simulink model "gm_sampleModel1933_1_sub"  (R2023a)
settings: Solver=VariableStepAuto  StartTime=0.0  StopTime=10.0  RelTol=1e-3
libraries: simulink x2
settings Model: Creator=user1  LastModifiedBy=user1
settings OptimizationCC: BlockReduction=off  ConditionallyExecuteInputs=off
settings DebuggingCC: InheritedTsInSrcMsg=none

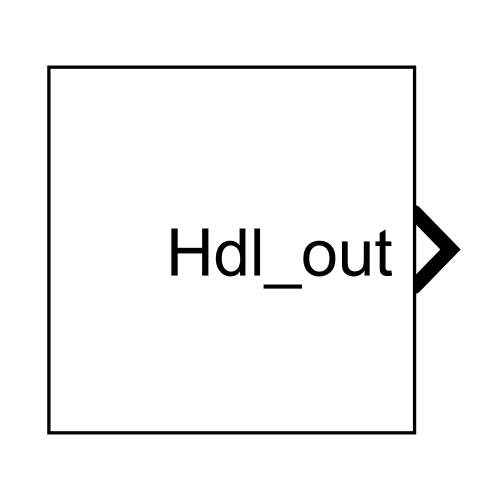
[thumbnail: Simulink's stored preview of the top-level diagram]
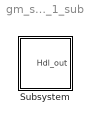
== system gm_sampleModel1933_1_sub ==
  Subsystem : Subsystem

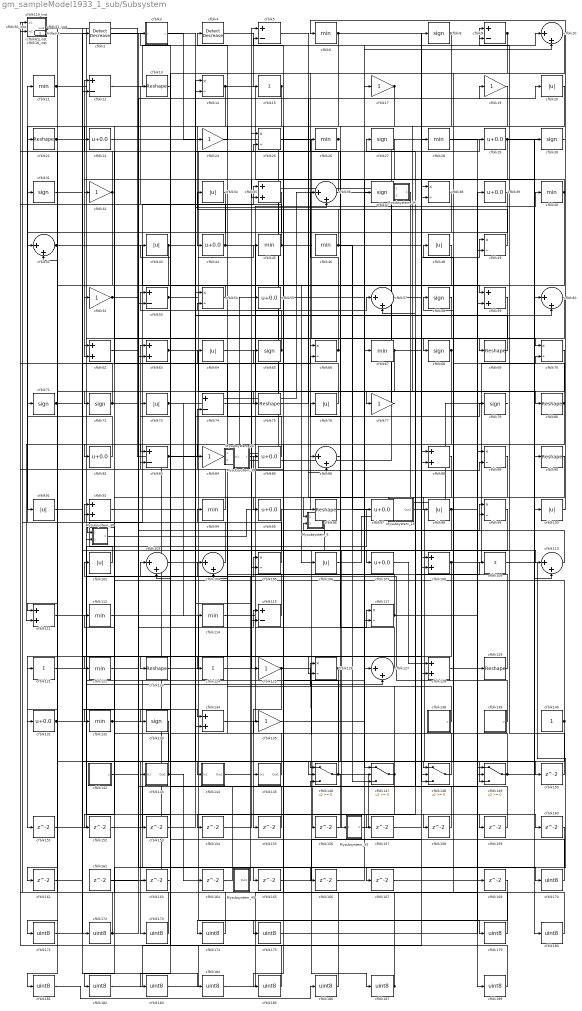
== system gm_sampleModel1933_1_sub/Subsystem ==
  Mysubsystem_13 : Subsystem
  Mysubsystem_24 : Subsystem
  Mysubsystem_30 : Subsystem
  Mysubsystem_33 : Subsystem
  Mysubsystem_34 : Subsystem
  Mysubsystem_39 : Subsystem
  Mysubsystem_45 : Subsystem
  Mysubsystem_9 : Subsystem
  cfblk{10,36,41,57,60,86,103..104,110,127} (10 alike) : Sum  Inputs=|++  OutDataTypeStr=uint8
  cfblk{20,34,43,48,64,73,76,91,98,100,102,106} (12 alike) : Abs  OutDataTypeStr=uint8  SaturateOnIntegerOverflow=off
  cfblk{14,25,38,49,54,66,70,89,99,105,117,126} (12 alike) : Product  Inputs=*/  OutDataTypeStr=uint8  RndMeth=Zero  SaturateOnIntegerOverflow=on
  cfblk{22,29,39,44,55,82,85,95,97,107,131} (11 alike) : Bias  Bias=0.0  SaturateOnIntegerOverflow=off
  cfblk{35,59,62..63,88,92,108,111,128,134} (10 alike) : Sum  OutDataTypeStr=uint8
  cfblk{15,109,121,124} (4 alike) : Sum  Inputs=+  OutDataTypeStr=uint8
  cfblk{6,11,26,28,40,45..46,67,94,112,114,122,132} (13 alike) : MinMax  OutDataTypeStr=uint8
  cfblk113_inst : Subsystem
  cfblk{5,9,12,53,74,83,115} (7 alike) : Sum  Inputs=+-  OutDataTypeStr=uint8
  cfblk119_inst : Subsystem
  cfblk{13,21,69,75,80,90,96,123,129} (9 alike) : Reshape
  cfblk{17,19,24,32,52,77,84,125,135} (9 alike) : Gain  OutDataTypeStr=uint8
  cfblk{8,27,30..31,37,58,65,68,71..72,79,133} (12 alike) : Signum
  cfblk138 : Subsystem  mask(Counter Free-Running){NumBits=double(16), tsamp=double(-1)}
      mask prompts: NumBits "Simulink:masks:NumberOfBits_MP"; tsamp "Simulink:masks:SampleTime_MP"
      mask help: Simulink:masks:CounterFreeRunning_MD
  cfblk139 : Subsystem  mask(Counter Limited){uplimit=double(7), tsamp=double(-1)}
      mask prompts: uplimit "Simulink:masks:UpperLimit_MP"; tsamp "Simulink:masks:SampleTime_MP"
      mask help: Simulink:masks:CounterLimited_MD
      mask init:
      | nbits = double(8);
      | tsamp = double(-1);
      | uplimit = double(7);
  cfblk140 : Constant  OutDataTypeStr=uint8  SampleTime=-1
  cfblk142 : Subsystem  mask(Counter Limited){uplimit=double(7), tsamp=double(-1)}
      mask prompts: uplimit "Simulink:masks:UpperLimit_MP"; tsamp "Simulink:masks:SampleTime_MP"
      mask help: Simulink:masks:CounterLimited_MD
      mask init:
      | nbits = double(8);
      | tsamp = double(-1);
      | uplimit = double(7);
  cfblk143 : Subsystem
  cfblk144 : Subsystem
  cfblk145 : Subsystem
  cfblk{146..149} (4 alike) : Switch  OutDataTypeStr=uint8  SaturateOnIntegerOverflow=off  InputSameDT=off
  cfblk{150..167,169} (19 alike) : Delay  SampleTime=1
  cfblk16_inst : Subsystem
  cfblk{170..175,179..187,189} (16 alike) : DataTypeConversion  OutDataTypeStr=uint8  SaturateOnIntegerOverflow=off  RndMeth=Floor
  cfblk2 : simulink/Logic and Bit Operations/Detect Decrease  vinit=0.0  OutDataTypeStr=uint8
      settings: LibrarySourceBlock=|
      | hdlsllib/Logic and Bit
      | Operations/Detect
      | Decrease
  cfblk3 : Subsystem  mask(Compare To Constant){relop=<=, const=double(3), OutDataTypeStr=uint8, ZeroCross=on}
      mask prompts: relop "Simulink:masks:Operator_MP"; const "Simulink:masks:ConstantValue_MP"; OutDataTypeStr "Simulink:masks:OutputDataType_MP"; ZeroCross "Simulink:masks:EnableZerocrossingDetection_MP"
      mask help: Simulink:masks:CompareToConstant_MD
      mask init:
      | OutDataTypeStr = 'uint8';
      | ZeroCross = 'on';
      | blkName = 'sampleModel1933_1_sub/Subsystem/cfblk3';
      | const = double(3);
      | const_str = '3.0';
      | const_val = double(3);
      | relop = '<=';
      | setValue = 'fixdt(0, 8)';
      | str = '<= 3';
      mask TypeOptions relop: == | ~= | < | <= | >= | >
      mask TypeOptions OutDataTypeStr: Simulink:masks:uint8 | Simulink:masks:boolean
      mask Callback ZeroCross: sl('zeroCrossEnable', gcbh);
      mask Display: disp(str)
  cfblk4 : simulink/Logic and Bit Operations/Detect Decrease  vinit=0.0  OutDataTypeStr=uint8
      settings: LibrarySourceBlock=|
      | hdlsllib/Logic and Bit
      | Operations/Detect
      | Decrease
  cfblk50_inst : Subsystem
  cfblk51_inst : Subsystem
  cfblk61_inst : Subsystem
  Hdl_out : Outport  OutDataTypeStr=uint8  SampleTime=1
  wires:
  Mysubsystem_13/1(Out1) -> cfblk150/1
  Mysubsystem_24/1(Out1) -> cfblk162/1
  Mysubsystem_30/1(Out1) -> Mysubsystem_13/2(In2)
  Mysubsystem_33/1(Out1) -> cfblk158/1
  Mysubsystem_34/1(Out1) -> Mysubsystem_9/1(In1)
  Mysubsystem_39/1(Y) -> cfblk57/1
  Mysubsystem_45/1(Out1) -> cfblk103/1
  Mysubsystem_9/1(Out1) -> Mysubsystem_33/1(In1)
  cfblk10/1 -> cfblk96/1
  cfblk100/1 -> cfblk6/1
  cfblk102/1 -> cfblk35/1
  cfblk103/1 -> cfblk187/1
  cfblk104/1 -> cfblk11/1
  cfblk105/1 -> cfblk16_inst/1(in1)
  cfblk106/1 -> Mysubsystem_13/3(In3)
  cfblk107/1 -> cfblk128/1
  cfblk108/1 -> cfblk70/2, cfblk151/1
  cfblk109/1 -> cfblk167/1
  cfblk11/1 -> cfblk128/2, cfblk127/2, cfblk159/1
  cfblk110/1 -> Mysubsystem_9/2(In2)
  cfblk111/1 -> cfblk123/1
  cfblk112/1 -> cfblk179/1
  cfblk113_inst/1(out1) -> cfblk68/1
  cfblk114/1 -> cfblk40/1
  cfblk115/1 -> cfblk51_inst/1(in1)
  cfblk117/1 -> cfblk63/1, cfblk189/1
  cfblk119_inst/1(out1) -> Mysubsystem_30/2(In2)
  cfblk12/1 -> cfblk10/1
  cfblk121/1 -> cfblk97/1
  cfblk122/1 -> cfblk99/1
  cfblk123/1 -> cfblk29/1
  cfblk124/1 -> cfblk117/1
  cfblk125/1 -> cfblk156/1, cfblk155/1
  cfblk126/1 -> cfblk173/1, cfblk161/1
  cfblk127/1 -> cfblk76/1
  cfblk128/1 -> cfblk59/2
  cfblk129/1 -> cfblk27/1
  cfblk13/1 -> cfblk163/1
  cfblk131/1 -> cfblk149/3, cfblk104/1, cfblk105/1
  cfblk132/1 -> cfblk37/1, cfblk165/1
  cfblk133/1 -> cfblk143/1(In1)
  cfblk134/1 -> cfblk109/1
  cfblk135/1 -> cfblk17/1
  cfblk138/1(y) -> cfblk126/1
  cfblk139/1(y) -> cfblk102/1
  cfblk14/1 -> cfblk127/1, cfblk110/2, cfblk122/1
  cfblk140/1 -> cfblk92/1, cfblk145/1(In1)
  cfblk142/1(y) -> cfblk115/1
  cfblk143/1(Out1) -> cfblk92/2, cfblk164/1
  cfblk144/1(Out1) -> cfblk89/2
  cfblk145/1(Out1) -> cfblk135/1
  cfblk146/1 -> cfblk25/2, cfblk160/1
  cfblk147/1 -> cfblk74/2, cfblk154/1
  cfblk148/1 -> cfblk94/1
  cfblk149/1 -> cfblk30/1, cfblk3/1(u)
  cfblk15/1 -> cfblk62/2, cfblk44/1, cfblk84/1
  cfblk150/1 -> cfblk9/1
  cfblk151/1 -> cfblk14/1
  cfblk152/1 -> cfblk108/1
  cfblk153/1 -> cfblk36/2
  cfblk154/1 -> cfblk99/2
  cfblk155/1 -> cfblk54/2
  cfblk156/1 -> cfblk147/2
  cfblk157/1 -> cfblk49/1
  cfblk158/1 -> cfblk83/2
  cfblk159/1 -> cfblk57/2
  cfblk16_inst/1(out1) -> cfblk108/2
  cfblk160/1 -> cfblk182/1
  cfblk161/1 -> cfblk66/2
  cfblk162/1 -> cfblk63/2
  cfblk163/1 -> cfblk53/1
  cfblk164/1 -> cfblk149/1
  cfblk165/1 -> cfblk88/2
  cfblk166/1 -> cfblk10/2
  cfblk167/1 -> cfblk89/1
  cfblk169/1 -> cfblk174/1
  cfblk17/1 -> cfblk91/1, cfblk86/1
  cfblk170/1 -> cfblk73/1
  cfblk171/1 -> cfblk2/1
  cfblk172/1 -> cfblk16_inst/2(in2), cfblk146/3, cfblk119_inst/2(in2)
  cfblk173/1 -> cfblk31/1
  cfblk174/1 -> cfblk113_inst/2(in2)
  cfblk175/1 -> cfblk169/1
  cfblk179/1 -> cfblk58/1
  cfblk180/1 -> cfblk112/1
  cfblk181/1 -> cfblk186/1
  cfblk182/1 -> cfblk38/1
  cfblk183/1 -> cfblk38/2
  cfblk184/1 -> cfblk49/2
  cfblk185/1 -> cfblk50_inst/1(in1)
  cfblk186/1 -> cfblk50_inst/2(in2)
  cfblk187/1 -> cfblk85/1, cfblk71/1, cfblk61_inst/1(in1)
  cfblk189/1 -> cfblk103/2
  cfblk19/1 -> cfblk75/1
  cfblk2/1 -> cfblk170/1
  cfblk20/1 -> cfblk24/1
  cfblk21/1 -> cfblk180/1, cfblk66/1
  cfblk22/1 -> cfblk110/1
  cfblk24/1 -> cfblk4/1
  cfblk25/1 -> cfblk59/1
  cfblk26/1 -> Hdl_out/1, Mysubsystem_24/1(In1)
  cfblk27/1 -> cfblk62/1
  cfblk28/1 -> cfblk80/1
  cfblk29/1 -> cfblk60/1, cfblk35/2
  cfblk3/1(y) -> cfblk115/2
  cfblk30/1 -> Mysubsystem_24/2(In2)
  cfblk31/1 -> cfblk172/1
  cfblk32/1 -> cfblk61_inst/2(in2), cfblk111/1
  cfblk34/1 -> cfblk131/1
  cfblk35/1 -> cfblk152/1
  cfblk36/1 -> cfblk12/1
  cfblk37/1 -> cfblk74/1
  cfblk38/1 -> cfblk181/1
  cfblk39/1 -> cfblk41/1
  cfblk4/1 -> cfblk15/1
  cfblk40/1 -> cfblk53/2, cfblk32/1
  cfblk41/1 -> cfblk148/3, cfblk106/1
  cfblk43/1 -> cfblk14/2, Mysubsystem_30/1(In1)
  cfblk44/1 -> cfblk113_inst/1(in1), cfblk117/2
  cfblk45/1 -> cfblk90/1, cfblk86/2, cfblk13/1
  cfblk46/1 -> cfblk5/2, cfblk147/3, cfblk28/1
  cfblk48/1 -> cfblk153/1
  cfblk49/1 -> cfblk34/1
  cfblk5/1 -> cfblk147/1
  cfblk50_inst/1(out1) -> cfblk184/1
  cfblk51_inst/1(out1) -> cfblk144/1(In1), Mysubsystem_39/1(In1)
  cfblk52/1 -> cfblk82/1, cfblk149/2
  cfblk53/1 -> cfblk146/1, cfblk45/1
  cfblk54/1 -> cfblk52/1
  cfblk55/1 -> cfblk67/1
  cfblk57/1 -> cfblk69/1
  cfblk58/1 -> cfblk72/1
  cfblk59/1 -> cfblk157/1
  cfblk6/1 -> cfblk88/1, cfblk171/1
  cfblk60/1 -> cfblk148/1
  cfblk61_inst/1(out1) -> cfblk41/2, cfblk126/2
  cfblk62/1 -> cfblk166/1
  cfblk63/1 -> cfblk100/1, cfblk70/1
  cfblk64/1 -> cfblk129/1
  cfblk65/1 -> cfblk5/1, cfblk43/1
  cfblk66/1 -> cfblk36/1, cfblk146/2
  cfblk67/1 -> cfblk8/1, cfblk105/2
  cfblk68/1 -> cfblk185/1, cfblk175/1
  cfblk69/1 -> cfblk54/1
  cfblk70/1 -> cfblk121/1
  cfblk71/1 -> cfblk134/1, cfblk107/1
  cfblk72/1 -> cfblk51_inst/2(in2), cfblk19/1
  cfblk73/1 -> Mysubsystem_34/1(In1), cfblk114/1
  cfblk74/1 -> cfblk125/1
  cfblk75/1 -> cfblk20/1
  cfblk76/1 -> cfblk22/1
  cfblk77/1 -> Mysubsystem_34/2(In2)
  cfblk79/1 -> Mysubsystem_13/1(In1)
  cfblk8/1 -> cfblk134/2, cfblk77/1
  cfblk80/1 -> cfblk48/1, cfblk111/2
  cfblk82/1 -> cfblk21/1
  cfblk83/1 -> cfblk65/1, cfblk60/2, cfblk25/1
  cfblk84/1 -> cfblk55/1
  cfblk85/1 -> cfblk64/1
  cfblk86/1 -> cfblk26/1
  cfblk88/1 -> cfblk132/1
  cfblk89/1 -> cfblk124/1
  cfblk9/1 -> cfblk98/1, cfblk83/1, cfblk148/2
  cfblk90/1 -> cfblk95/1
  cfblk91/1 -> cfblk12/2
  cfblk92/1 -> cfblk79/1
  cfblk94/1 -> cfblk119_inst/1(in1)
  cfblk95/1 -> cfblk133/1
  cfblk96/1 -> cfblk9/2
  cfblk97/1 -> cfblk46/1
  cfblk98/1 -> cfblk39/1, cfblk104/2
  cfblk99/1 -> cfblk183/1

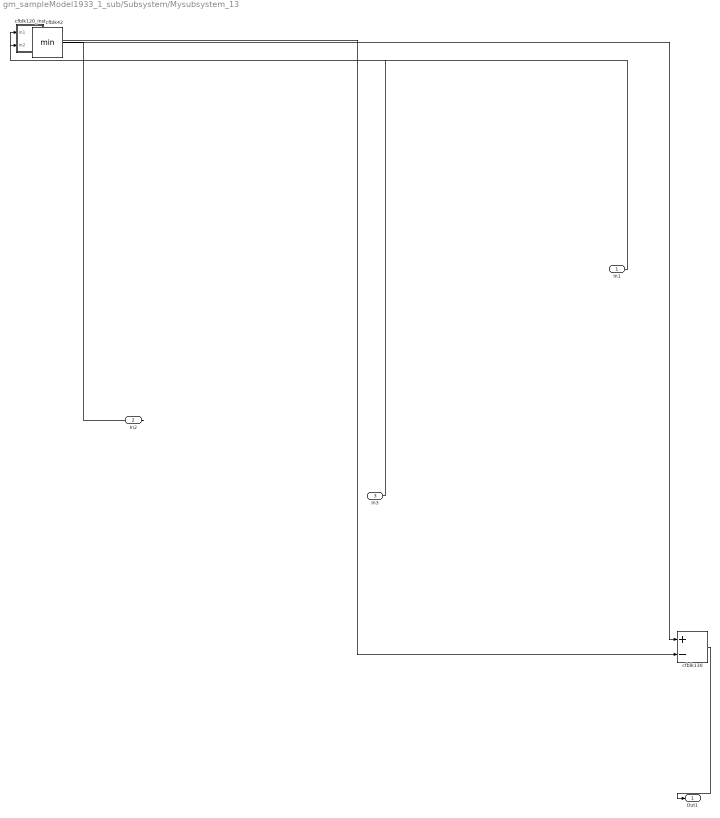
== system gm_sampleModel1933_1_sub/Subsystem/Mysubsystem_13 ==
  In1 : Inport  OutDataTypeStr=uint8  PortDimensions=1  SampleTime=1
  In2 : Inport  Port=2  OutDataTypeStr=uint8  PortDimensions=1  SampleTime=1
  In3 : Inport  Port=3  OutDataTypeStr=uint8  PortDimensions=1  SampleTime=1
  cfblk120_inst : Subsystem
  cfblk130 : Sum  Inputs=+-
  cfblk42 : MinMax
  Out1 : Outport  SampleTime=1
  wires:
  In1/1 -> cfblk120_inst/1(in1)
  In2/1 -> cfblk42/1
  In3/1 -> cfblk120_inst/2(in2)
  cfblk120_inst/1(out1) -> cfblk130/2
  cfblk130/1 -> Out1/1
  cfblk42/1 -> cfblk130/1

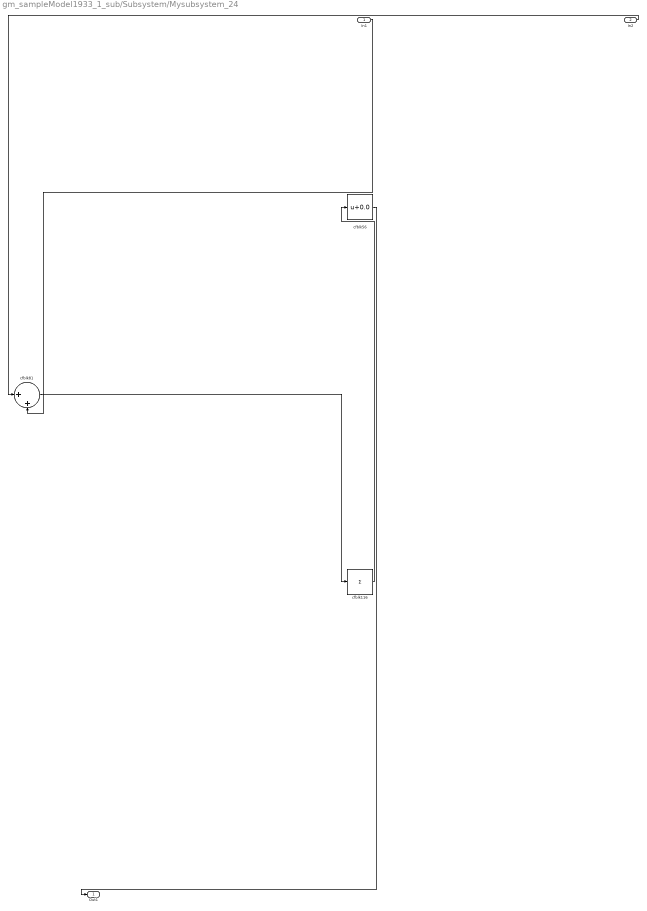
== system gm_sampleModel1933_1_sub/Subsystem/Mysubsystem_24 ==
  In1 : Inport  OutDataTypeStr=uint8  PortDimensions=1  SampleTime=1
  In2 : Inport  Port=2  OutDataTypeStr=uint8  PortDimensions=1  SampleTime=1
  cfblk116 : Sum  Inputs=+
  cfblk56 : Bias  Bias=0.0  SaturateOnIntegerOverflow=off
  cfblk81 : Sum  Inputs=|++
  Out1 : Outport  SampleTime=1
  wires:
  In1/1 -> cfblk81/2
  In2/1 -> cfblk81/1
  cfblk116/1 -> cfblk56/1
  cfblk56/1 -> Out1/1
  cfblk81/1 -> cfblk116/1

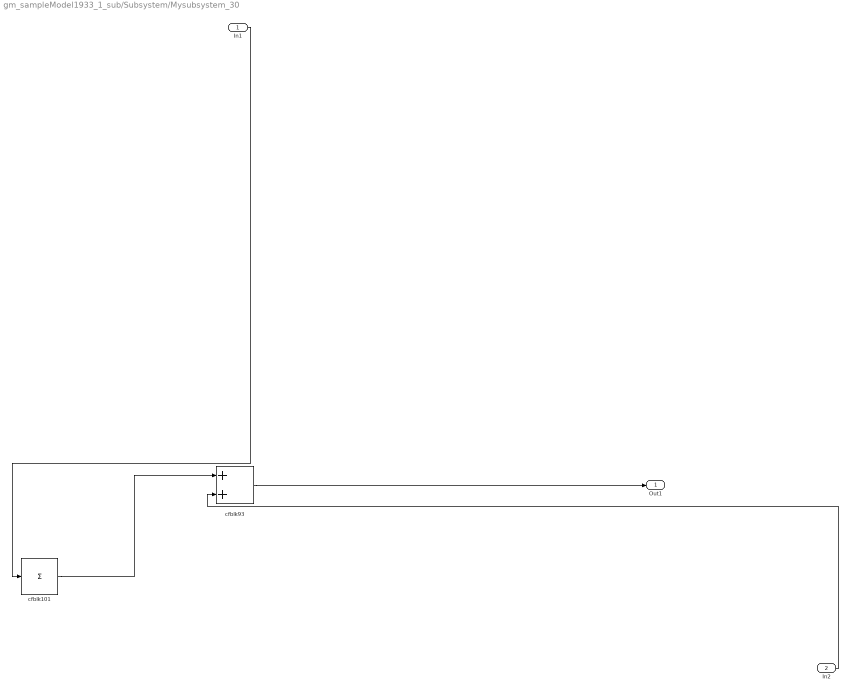
== system gm_sampleModel1933_1_sub/Subsystem/Mysubsystem_30 ==
  In1 : Inport  OutDataTypeStr=uint8  PortDimensions=1  SampleTime=1
  In2 : Inport  Port=2  OutDataTypeStr=uint8  PortDimensions=1  SampleTime=1
  cfblk101 : Sum  Inputs=+
  cfblk93 : Sum
  Out1 : Outport  SampleTime=1
  wires:
  In1/1 -> cfblk101/1
  In2/1 -> cfblk93/2
  cfblk101/1 -> cfblk93/1
  cfblk93/1 -> Out1/1

== system gm_sampleModel1933_1_sub/Subsystem/Mysubsystem_33 ==
  In1 : Inport  OutDataTypeStr=uint16  PortDimensions=1  SampleTime=1
  cfblk176 : DataTypeConversion  SaturateOnIntegerOverflow=off  RndMeth=Floor
  Out1 : Outport  SampleTime=1
  wires:
  In1/1 -> cfblk176/1
  cfblk176/1 -> Out1/1

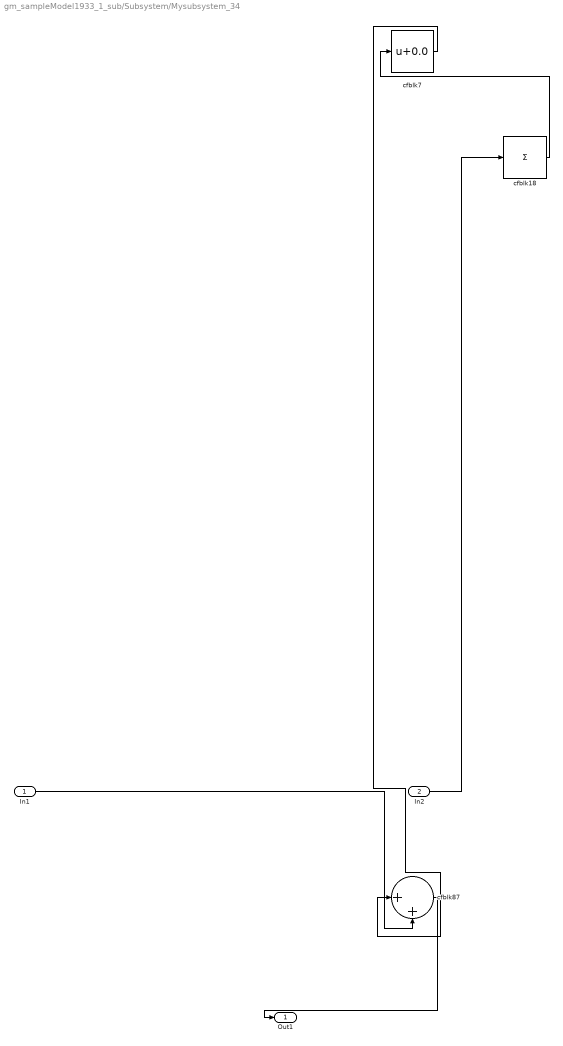
== system gm_sampleModel1933_1_sub/Subsystem/Mysubsystem_34 ==
  In1 : Inport  OutDataTypeStr=uint8  PortDimensions=1  SampleTime=1
  In2 : Inport  Port=2  OutDataTypeStr=uint8  PortDimensions=1  SampleTime=1
  cfblk18 : Sum  Inputs=+
  cfblk7 : Bias  Bias=0.0  SaturateOnIntegerOverflow=off
  cfblk87 : Sum  Inputs=|++
  Out1 : Outport  SampleTime=1
  wires:
  In1/1 -> cfblk87/2
  In2/1 -> cfblk18/1
  cfblk18/1 -> cfblk7/1
  cfblk7/1 -> cfblk87/1
  cfblk87/1 -> Out1/1

== system gm_sampleModel1933_1_sub/Subsystem/Mysubsystem_39 ==
  In1 : Inport  OutDataTypeStr=uint8  PortDimensions=1  SampleTime=1
  cfblk1 : Subsystem  mask(Detect Rise Positive){vinit=double(0), InputProcessing=Elements as channels (sample based), OutDataTypeStr=boolean}
      mask prompts: vinit "Simulink:masks:InitialCondition_MP"; InputProcessing "Simulink:masks:InputProcessing_MP"; OutDataTypeStr "Simulink:masks:OutputDataType_MP"
      mask help: Simulink:masks:DetectRisePositive_MD
      mask init:
      | InputProcessing = 'Elements as channels (sample based)';
      | OutDataTypeStr = 'boolean';
      | vinit = double(0);
      mask TypeOptions InputProcessing: Simulink:masks:ColumnsAsChannelsFrameBased | Simulink:masks:ElementsAsChannelsSampleBased
      mask TypeOptions OutDataTypeStr: Simulink:masks:uint8 | Simulink:masks:boolean
      mask Display: fprintf('U > 0\n&  NOT\nU/z > 0')
  cfblk168 : Delay  SampleTime=1
  Y : Outport  SampleTime=1
  wires:
  In1/1 -> cfblk168/1
  cfblk1/1(Y) -> Y/1
  cfblk168/1 -> cfblk1/1(U)

== system gm_sampleModel1933_1_sub/Subsystem/Mysubsystem_45 ==
  cfblk141 : Ground
  cfblk188 : DataTypeConversion  OutDataTypeStr=uint8  SaturateOnIntegerOverflow=off  RndMeth=Floor
  Out1 : Outport  SampleTime=1
  wires:
  cfblk141/1 -> cfblk188/1
  cfblk188/1 -> Out1/1

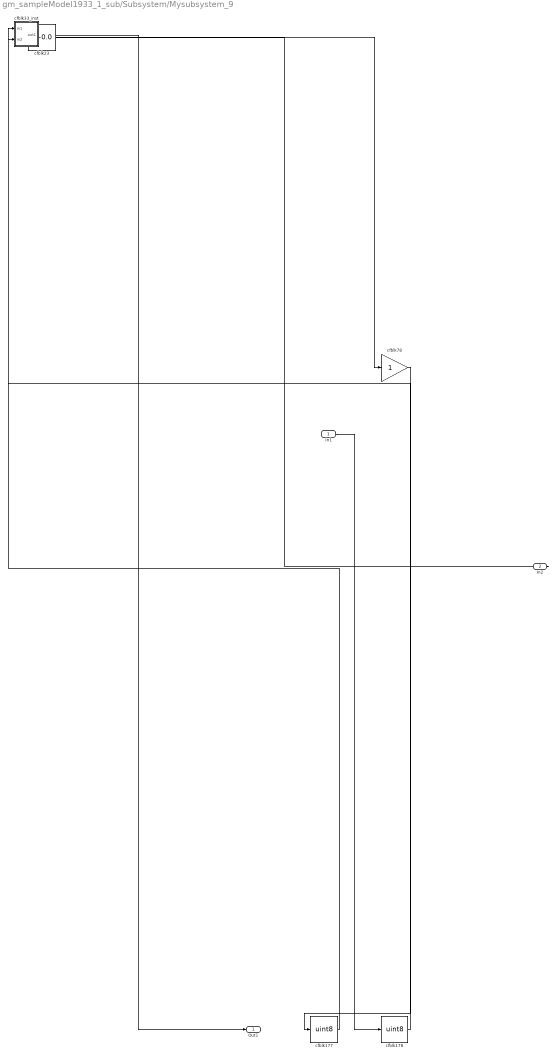
== system gm_sampleModel1933_1_sub/Subsystem/Mysubsystem_9 ==
  In1 : Inport  OutDataTypeStr=uint8  PortDimensions=1  SampleTime=1
  In2 : Inport  Port=2  OutDataTypeStr=uint8  PortDimensions=1  SampleTime=1
  cfblk177 : DataTypeConversion  OutDataTypeStr=uint8  SaturateOnIntegerOverflow=off  RndMeth=Floor
  cfblk178 : DataTypeConversion  OutDataTypeStr=uint8  SaturateOnIntegerOverflow=off  RndMeth=Floor
  cfblk23 : Bias  Bias=0.0  SaturateOnIntegerOverflow=off
  cfblk33_inst : Subsystem
  cfblk78 : Gain
  Out1 : Outport  SampleTime=1
  wires:
  In1/1 -> cfblk178/1
  In2/1 -> cfblk23/1
  cfblk177/1 -> cfblk33_inst/1(in1)
  cfblk178/1 -> cfblk33_inst/2(in2)
  cfblk23/1 -> cfblk78/1
  cfblk33_inst/1(out1) -> Out1/1
  cfblk78/1 -> cfblk177/1

== system gm_sampleModel1933_1_sub/Subsystem/cfblk113_inst ==
  in1 : Inport  OutDataTypeStr=uint8  SampleTime=1
  in2 : Inport  Port=2  OutDataTypeStr=uint8  SampleTime=1
  mul_cfblk113_dotp_mulcomp : Product  Inputs=**  OutDataTypeStr=uint8  SampleTime=1
  out1 : Outport  OutDataTypeStr=uint8  SampleTime=1
  wires:
  in1/1 -> mul_cfblk113_dotp_mulcomp/1
  in2/1 -> mul_cfblk113_dotp_mulcomp/2
  mul_cfblk113_dotp_mulcomp/1 -> out1/1

== system gm_sampleModel1933_1_sub/Subsystem/cfblk119_inst ==
  in1 : Inport  OutDataTypeStr=uint8  SampleTime=1
  in2 : Inport  Port=2  OutDataTypeStr=uint8  SampleTime=1
  mul_cfblk119_dotp_mulcomp : Product  Inputs=**  OutDataTypeStr=uint8  SampleTime=1
  out1 : Outport  OutDataTypeStr=uint8  SampleTime=1
  wires:
  in1/1 -> mul_cfblk119_dotp_mulcomp/1
  in2/1 -> mul_cfblk119_dotp_mulcomp/2
  mul_cfblk119_dotp_mulcomp/1 -> out1/1

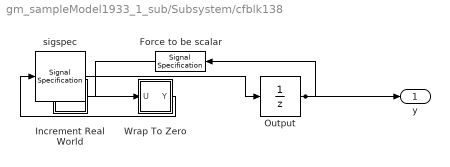
== system gm_sampleModel1933_1_sub/Subsystem/cfblk138 ==
  Force to be scalar : SignalSpecification  DisableCoverage=on  Dimensions=1
  Increment Real World : Subsystem  mask(Real World Value Increment){}
      mask help: Simulink:masks:RealWorldValueIncrement_MD
      mask Display: disp('V++')
  Output : UnitDelay  InitialCondition=0.0  SampleTime=tsamp  HasFrameUpgradeWarning=on
  Wrap To Zero : Subsystem  mask(Wrap To Zero){Threshold=double(65535)}
      mask prompts: Threshold "Simulink:masks:Threshold_MP"
      mask help: Simulink:masks:WrapToZero_MD
  sigspec : SignalSpecification  OutDataTypeStr=uint16  Dimensions=1
  y : Outport  SampleTime=1
  wires:
  Force to be scalar/1 -> Increment Real World/1(u)
  Increment Real World/1(y) -> Wrap To Zero/1(U)
  Output/1 -> Force to be scalar/1, y/1
  Wrap To Zero/1(Y) -> sigspec/1
  sigspec/1 -> Output/1

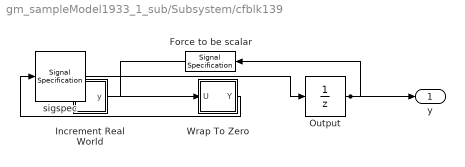
== system gm_sampleModel1933_1_sub/Subsystem/cfblk139 ==
  Force to be scalar : SignalSpecification  DisableCoverage=on  Dimensions=1
  Increment Real World : Subsystem  mask(Real World Value Increment){}
      mask help: Simulink:masks:RealWorldValueIncrement_MD
      mask Display: disp('V++')
  Output : UnitDelay  InitialCondition=0.0  SampleTime=tsamp  HasFrameUpgradeWarning=on
  Wrap To Zero : Subsystem  mask(Wrap To Zero){Threshold=double(7)}
      mask prompts: Threshold "Simulink:masks:Threshold_MP"
      mask help: Simulink:masks:WrapToZero_MD
  sigspec : SignalSpecification  OutDataTypeStr=uint8  Dimensions=1
  y : Outport  SampleTime=1
  wires:
  Force to be scalar/1 -> Increment Real World/1(u)
  Increment Real World/1(y) -> Wrap To Zero/1(U)
  Output/1 -> Force to be scalar/1, y/1
  Wrap To Zero/1(Y) -> sigspec/1
  sigspec/1 -> Output/1

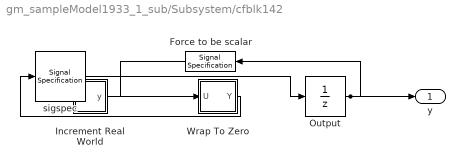
== system gm_sampleModel1933_1_sub/Subsystem/cfblk142 ==
  Force to be scalar : SignalSpecification  DisableCoverage=on  Dimensions=1
  Increment Real World : Subsystem  mask(Real World Value Increment){}
      mask help: Simulink:masks:RealWorldValueIncrement_MD
      mask Display: disp('V++')
  Output : UnitDelay  InitialCondition=0.0  SampleTime=tsamp  HasFrameUpgradeWarning=on
  Wrap To Zero : Subsystem  mask(Wrap To Zero){Threshold=double(7)}
      mask prompts: Threshold "Simulink:masks:Threshold_MP"
      mask help: Simulink:masks:WrapToZero_MD
  sigspec : SignalSpecification  OutDataTypeStr=uint8  Dimensions=1
  y : Outport  SampleTime=1
  wires:
  Force to be scalar/1 -> Increment Real World/1(u)
  Increment Real World/1(y) -> Wrap To Zero/1(U)
  Output/1 -> Force to be scalar/1, y/1
  Wrap To Zero/1(Y) -> sigspec/1
  sigspec/1 -> Output/1

== system gm_sampleModel1933_1_sub/Subsystem/cfblk143 ==
  In1 : Inport  OutDataTypeStr=uint8  PortDimensions=1  SampleTime=1
  Out1 : Outport  SampleTime=1
  wires:
  In1/1 -> Out1/1

== system gm_sampleModel1933_1_sub/Subsystem/cfblk144 ==
  In1 : Inport  OutDataTypeStr=uint8  PortDimensions=1  SampleTime=1
  Out1 : Outport  SampleTime=1
  wires:
  In1/1 -> Out1/1

== system gm_sampleModel1933_1_sub/Subsystem/cfblk145 ==
  In1 : Inport  OutDataTypeStr=uint8  PortDimensions=1  SampleTime=1
  Out1 : Outport  SampleTime=1
  wires:
  In1/1 -> Out1/1

== system gm_sampleModel1933_1_sub/Subsystem/cfblk16_inst ==
  in1 : Inport  OutDataTypeStr=uint8  SampleTime=1
  in2 : Inport  Port=2  OutDataTypeStr=uint8  SampleTime=1
  mul_cfblk16_dotp_mulcomp : Product  Inputs=**  OutDataTypeStr=uint8  SampleTime=1
  out1 : Outport  OutDataTypeStr=uint8  SampleTime=1
  wires:
  in1/1 -> mul_cfblk16_dotp_mulcomp/1
  in2/1 -> mul_cfblk16_dotp_mulcomp/2
  mul_cfblk16_dotp_mulcomp/1 -> out1/1

== system gm_sampleModel1933_1_sub/Subsystem/cfblk3 ==
  u : Inport  OutDataTypeStr=uint8  SampleTime=1
  Compare : RelationalOperator  Operator=<=  OutDataTypeStr=fixdt(0, 8)
  Constant : Constant  DisableCoverage=on  Value=const  OutDataTypeStr=Inherit: Inherit via back propagation  SampleTime=-1
  y : Outport  SampleTime=1
  wires:
  u/1 -> Compare/1
  Compare/1 -> y/1
  Constant/1 -> Compare/2

== system gm_sampleModel1933_1_sub/Subsystem/cfblk50_inst ==
  in1 : Inport  OutDataTypeStr=uint8  SampleTime=1
  in2 : Inport  Port=2  OutDataTypeStr=uint8  SampleTime=1
  mul_cfblk50_dotp_mulcomp : Product  Inputs=**  OutDataTypeStr=uint8  SampleTime=1
  out1 : Outport  OutDataTypeStr=uint8  SampleTime=1
  wires:
  in1/1 -> mul_cfblk50_dotp_mulcomp/1
  in2/1 -> mul_cfblk50_dotp_mulcomp/2
  mul_cfblk50_dotp_mulcomp/1 -> out1/1

== system gm_sampleModel1933_1_sub/Subsystem/cfblk51_inst ==
  in1 : Inport  OutDataTypeStr=uint8  SampleTime=1
  in2 : Inport  Port=2  OutDataTypeStr=uint8  SampleTime=1
  mul_cfblk51_dotp_mulcomp : Product  Inputs=**  OutDataTypeStr=uint8  SampleTime=1
  out1 : Outport  OutDataTypeStr=uint8  SampleTime=1
  wires:
  in1/1 -> mul_cfblk51_dotp_mulcomp/1
  in2/1 -> mul_cfblk51_dotp_mulcomp/2
  mul_cfblk51_dotp_mulcomp/1 -> out1/1

== system gm_sampleModel1933_1_sub/Subsystem/cfblk61_inst ==
  in1 : Inport  OutDataTypeStr=uint8  SampleTime=1
  in2 : Inport  Port=2  OutDataTypeStr=uint8  SampleTime=1
  mul_cfblk61_dotp_mulcomp : Product  Inputs=**  OutDataTypeStr=uint8  SampleTime=1
  out1 : Outport  OutDataTypeStr=uint8  SampleTime=1
  wires:
  in1/1 -> mul_cfblk61_dotp_mulcomp/1
  in2/1 -> mul_cfblk61_dotp_mulcomp/2
  mul_cfblk61_dotp_mulcomp/1 -> out1/1

== system gm_sampleModel1933_1_sub/Subsystem/Mysubsystem_13/cfblk120_inst ==
  in1 : Inport  OutDataTypeStr=uint8  SampleTime=1
  in2 : Inport  Port=2  OutDataTypeStr=uint8  SampleTime=1
  mul_cfblk120_dotp_mulcomp : Product  Inputs=**  OutDataTypeStr=uint16  SampleTime=1
  out1 : Outport  OutDataTypeStr=uint16  SampleTime=1
  wires:
  in1/1 -> mul_cfblk120_dotp_mulcomp/1
  in2/1 -> mul_cfblk120_dotp_mulcomp/2
  mul_cfblk120_dotp_mulcomp/1 -> out1/1

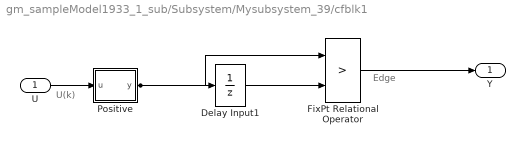
== system gm_sampleModel1933_1_sub/Subsystem/Mysubsystem_39/cfblk1 ==
  note: U(k)
  note: Edge
  U : Inport  OutDataTypeStr=uint8  SampleTime=1
  Delay Input1 : UnitDelay  Description=Store in Global RAM  DisableCoverage=on  InitialCondition=vinit  SampleTime=-1  HasFrameUpgradeWarning=on
  FixPt Relational Operator : RelationalOperator  Operator=>  OutDataTypeStr=boolean  ZeroCross=off  InputSameDT=off
  Positive : Subsystem  mask(Compare To Zero){relop=>, OutDataTypeStr=boolean, ZeroCross=off}
      mask prompts: relop "Simulink:masks:Operator_MP"; OutDataTypeStr "Simulink:masks:OutputDataType_MP"; ZeroCross "Simulink:masks:EnableZerocrossingDetection_MP"
      mask help: Simulink:masks:CompareToZero_MD
      mask init:
      | OutDataTypeStr = 'boolean';
      | ZeroCross = 'off';
      | blkName = 'sampleModel1933_1_sub/Subsystem/Mysubsystem_39/cfblk1/Positive';
      | relop = '>';
      | setValue = 'boolean';
      mask TypeOptions relop: == | ~= | < | <= | >= | >
      mask TypeOptions OutDataTypeStr: Simulink:masks:uint8 | Simulink:masks:boolean
      mask Callback ZeroCross: sl('zeroCrossEnable', gcbh);
      mask Display: disp([relop,' 0'])
  Y : Outport  SampleTime=1
  wires:
  U/1 -> Positive/1(u)
  Delay Input1/1 -> FixPt Relational Operator/2
  FixPt Relational Operator/1 -> Y/1
  Positive/1(y) -> FixPt Relational Operator/1, Delay Input1/1

== system gm_sampleModel1933_1_sub/Subsystem/Mysubsystem_9/cfblk33_inst ==
  in1 : Inport  OutDataTypeStr=uint8  SampleTime=1
  in2 : Inport  Port=2  OutDataTypeStr=uint8  SampleTime=1
  mul_cfblk33_dotp_mulcomp : Product  Inputs=**  OutDataTypeStr=uint16  SampleTime=1
  out1 : Outport  OutDataTypeStr=uint16  SampleTime=1
  wires:
  in1/1 -> mul_cfblk33_dotp_mulcomp/1
  in2/1 -> mul_cfblk33_dotp_mulcomp/2
  mul_cfblk33_dotp_mulcomp/1 -> out1/1

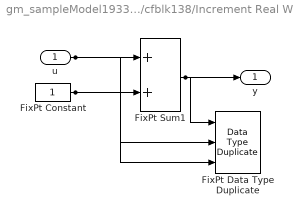
== system gm_sampleModel1933_1_sub/Subsystem/cfblk138/Increment Real World ==
  u : Inport  OutDataTypeStr=uint16  SampleTime=1
  FixPt Constant : Constant  DisableCoverage=on  OutDataTypeStr=Inherit: Inherit via back propagation  SampleTime=-1
  FixPt Data Type Duplicate : DataTypeDuplicate  DisableCoverage=on  NumInputPorts=3
  FixPt Sum1 : Sum  InputSameDT=on  OutDataTypeStr=Inherit: Inherit via back propagation  LockScale=on
  y : Outport  SampleTime=1
  wires:
  u/1 -> FixPt Sum1/1, FixPt Data Type Duplicate/2
  FixPt Constant/1 -> FixPt Sum1/2, FixPt Data Type Duplicate/3
  FixPt Sum1/1 -> FixPt Data Type Duplicate/1, y/1

== system gm_sampleModel1933_1_sub/Subsystem/cfblk138/Wrap To Zero ==
  note: U(k)
  U : Inport  OutDataTypeStr=uint16  SampleTime=1
  Constant : Constant  DisableCoverage=on  Value=0  OutDataTypeStr=Inherit: Inherit via back propagation  SampleTime=-1
  FixPt Data Type Duplicate1 : DataTypeDuplicate  DisableCoverage=on  NumInputPorts=3
  FixPt Switch : Switch  Criteria=u2 > Threshold  Threshold=Threshold  OutDataTypeStr=Inherit: Inherit via back propagation  ZeroCross=off  SaturateOnIntegerOverflow=off  InputSameDT=off
  Y : Outport  SampleTime=1
  wires:
  U/1 -> FixPt Switch/3, FixPt Switch/2, FixPt Data Type Duplicate1/2
  Constant/1 -> FixPt Switch/1, FixPt Data Type Duplicate1/3
  FixPt Switch/1 -> FixPt Data Type Duplicate1/1, Y/1

== system gm_sampleModel1933_1_sub/Subsystem/cfblk139/Increment Real World ==
  u : Inport  OutDataTypeStr=uint8  SampleTime=1
  FixPt Constant : Constant  DisableCoverage=on  OutDataTypeStr=Inherit: Inherit via back propagation  SampleTime=-1
  FixPt Data Type Duplicate : DataTypeDuplicate  DisableCoverage=on  NumInputPorts=3
  FixPt Sum1 : Sum  InputSameDT=on  OutDataTypeStr=Inherit: Inherit via back propagation  LockScale=on
  y : Outport  SampleTime=1
  wires:
  u/1 -> FixPt Sum1/1, FixPt Data Type Duplicate/2
  FixPt Constant/1 -> FixPt Sum1/2, FixPt Data Type Duplicate/3
  FixPt Sum1/1 -> FixPt Data Type Duplicate/1, y/1

== system gm_sampleModel1933_1_sub/Subsystem/cfblk139/Wrap To Zero ==
  note: U(k)
  U : Inport  OutDataTypeStr=uint8  SampleTime=1
  Constant : Constant  DisableCoverage=on  Value=0  OutDataTypeStr=Inherit: Inherit via back propagation  SampleTime=-1
  FixPt Data Type Duplicate1 : DataTypeDuplicate  DisableCoverage=on  NumInputPorts=3
  FixPt Switch : Switch  Criteria=u2 > Threshold  Threshold=Threshold  OutDataTypeStr=Inherit: Inherit via back propagation  ZeroCross=off  SaturateOnIntegerOverflow=off  InputSameDT=off
  Y : Outport  SampleTime=1
  wires:
  U/1 -> FixPt Switch/3, FixPt Switch/2, FixPt Data Type Duplicate1/2
  Constant/1 -> FixPt Switch/1, FixPt Data Type Duplicate1/3
  FixPt Switch/1 -> FixPt Data Type Duplicate1/1, Y/1

== system gm_sampleModel1933_1_sub/Subsystem/cfblk142/Increment Real World ==
  u : Inport  OutDataTypeStr=uint8  SampleTime=1
  FixPt Constant : Constant  DisableCoverage=on  OutDataTypeStr=Inherit: Inherit via back propagation  SampleTime=-1
  FixPt Data Type Duplicate : DataTypeDuplicate  DisableCoverage=on  NumInputPorts=3
  FixPt Sum1 : Sum  InputSameDT=on  OutDataTypeStr=Inherit: Inherit via back propagation  LockScale=on
  y : Outport  SampleTime=1
  wires:
  u/1 -> FixPt Sum1/1, FixPt Data Type Duplicate/2
  FixPt Constant/1 -> FixPt Sum1/2, FixPt Data Type Duplicate/3
  FixPt Sum1/1 -> FixPt Data Type Duplicate/1, y/1

== system gm_sampleModel1933_1_sub/Subsystem/cfblk142/Wrap To Zero ==
  note: U(k)
  U : Inport  OutDataTypeStr=uint8  SampleTime=1
  Constant : Constant  DisableCoverage=on  Value=0  OutDataTypeStr=Inherit: Inherit via back propagation  SampleTime=-1
  FixPt Data Type Duplicate1 : DataTypeDuplicate  DisableCoverage=on  NumInputPorts=3
  FixPt Switch : Switch  Criteria=u2 > Threshold  Threshold=Threshold  OutDataTypeStr=Inherit: Inherit via back propagation  ZeroCross=off  SaturateOnIntegerOverflow=off  InputSameDT=off
  Y : Outport  SampleTime=1
  wires:
  U/1 -> FixPt Switch/3, FixPt Switch/2, FixPt Data Type Duplicate1/2
  Constant/1 -> FixPt Switch/1, FixPt Data Type Duplicate1/3
  FixPt Switch/1 -> FixPt Data Type Duplicate1/1, Y/1

== system gm_sampleModel1933_1_sub/Subsystem/Mysubsystem_39/cfblk1/Positive ==
  u : Inport  OutDataTypeStr=uint8  SampleTime=1
  Compare : RelationalOperator  Operator=>  OutDataTypeStr=boolean  ZeroCross=off
  Constant : Constant  DisableCoverage=on  Value=0  OutDataTypeStr=Inherit: Inherit via back propagation  SampleTime=-1  PreserveConstantTs=on
  y : Outport  SampleTime=1
  wires:
  u/1 -> Compare/1
  Compare/1 -> y/1
  Constant/1 -> Compare/2
